simulink model "Original_id_ad28d30db84132bde97d93811f6c005a2439af74"  (R2020a)
settings: Solver=VariableStepAuto  StartTime=0.0  StopTime=10.0  RelTol=1e-3
model workspace (MAT data in the model file):
  InputValues_20210821T203440345 = [-1 -0.9921875 -0.984375 -0.9765625 -0.96875 -0.9609375 -0.953125 -0.9453125 -0.9375 -0.9296875 -0.921875 -0.9140625 ... (256 elements, 256x1)]
settings Model: Creator=Mahsa  LastModifiedBy=Mahsa

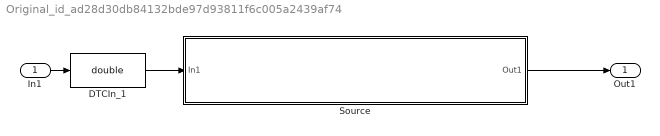
== system Original_id_ad28d30db84132bde97d93811f6c005a2439af74 ==
  In1 : Inport  OutDataTypeStr=fixdt(1,8,7)
  DTCIn_1 : DataTypeConversion  OutDataTypeStr=double  RndMeth=Nearest
  Source : Subsystem
      mask Display: fprintf('%s','tanh')
  Out1 : Outport
  wires:
  In1/1 -> DTCIn_1/1
  DTCIn_1/1 -> Source/1(In1)
  Source/1(Out1) -> Out1/1

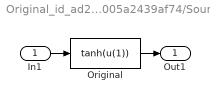
== system Original_id_ad28d30db84132bde97d93811f6c005a2439af74/Source ==
  In1 : Inport
  Original : MATLABFcn  MATLABFcn=tanh(u(1))
  Out1 : Outport
  wires:
  In1/1 -> Original/1
  Original/1 -> Out1/1
